simulink model "F16_openloop_linearization"  (R2018b)
settings: Solver=ode4  StartTime=0.0  StopTime=100.0  FixedStep=0.1  RelTol=1e-3  EnableMultiTasking=on
values from neighbouring files (symbols this model uses):
  fi_flag_Simulink = 0    [FindF16Dynamics.m]    (also in runF16model.m = 1)
libraries: simulink_extras x1
settings Model: Creator=Administrator  LastModifiedBy=LXS
settings DataIOCC: ExternalInput=[0 0.235629886402192 -0.0257557884830845 -0.00060101434994637 0.0105189516288919]  InitialState=[]  LimitDataPoints=on  LoadExternalInput=on  LoadInitialState=on  SaveFormat=Array  SignalLoggingSaveFormat=ModelDataLogs  SignalLoggingName=sigsOut
settings OptimizationCC: DefaultParameterBehavior=Inlined  BufferReuse=off  ExpressionDepthLimit=2147483647  InitFltsAndDblsToZero=on  LifeSpan=inf
settings DebuggingCC: SaveWithParameterizedLinksMsg=none  UnderspecifiedInitializationDetection=Classic  MergeDetectMultiDrivingBlocksExec=none  SignalResolutionControl=TryResolveAllWithWarning  MultiTaskDSMMsg=warning  MultiTaskCondExecSysMsg=none  FcnCallInpInsideContextMsg=warning  StateNameClashWarn=warning  InitInArrayFormatMsg=none  SFUnexpectedBacktrackingDiag=warning  SFNoUnconditionalDefaultTransitionDiag=warning  SFExecutionAtInitializationDiag=none
settings HardwareCC: ProdBitPerPointer=32  ProdBitPerSizeT=32  ProdBitPerPtrDiffT=32  ProdLargestAtomicFloat=None  ProdIntDivRoundTo=Undefined  ProdEndianess=Unspecified  ProdWordSize=32  ProdHWDeviceType=32-bit Generic  TargetUnknown=on
settings ModelReferenceCC: PropagateSignalLabelsOutOfModel=off
settings SFSimCC: SimUseLocalCustomCode=off
settings RTWCC: RTWUseLocalCustomCode=off
settings CodeAppCC: StateflowObjectComments=on
settings GRTTargetCC: TargetFcnLib=ansi_tfl_tmw.mat  TargetLangStandard=C89/C90 (ANSI)  GeneratePreprocessorConditionals=Disable all  CombineOutputUpdateFcns=off  GRTInterface=on
settings ConfigComp: CovMetricSettings=dw  CovHtmlReporting=on  CovSaveCumulativeToWorkspaceVar=on  CovSaveSingleToWorkspaceVar=on  CovExternalEMLEnable=off  CovSFcnEnable=off

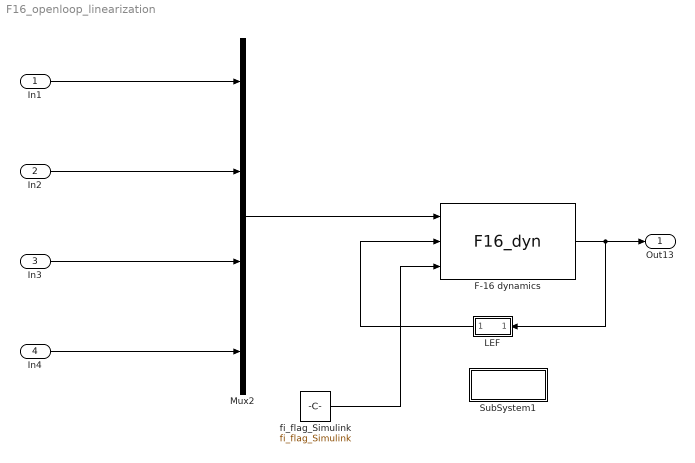
== system F16_openloop_linearization ==
  In1 : Inport
  In2 : Inport  Port=2
  In3 : Inport  Port=3
  In4 : Inport  Port=4
  F-16 dynamics : S-Function  FunctionName=F16_dyn  Parameters=init_x  SFunctionDeploymentMode=off  EnableBusSupport=off
      mask Display: image(imread('f16.jpg'))
  LEF : Subsystem
      mask Display: port_label('output', 1, 'dlef')
  Mux2 : Mux
  SubSystem1 : Subsystem
      settings: OpenFcn=edit(fullfile(cd,'F16_dyn.c'))
      mask Display: disp('F16_dyn.c');
  fi_flag_Simulink : Constant  Value=fi_flag_Simulink
  Out13 : Outport
  wires:
  F-16 dynamics/1 -> Out13/1, LEF/1(state)
  fi_flag_Simulink/1 -> F-16 dynamics/3
  LEF/1("delta_lef ") -> F-16 dynamics/2
  Mux2/1 -> F-16 dynamics/1
  In2/1 -> Mux2/2
  In3/1 -> Mux2/3
  In4/1 -> Mux2/4
  In1/1 -> Mux2/1

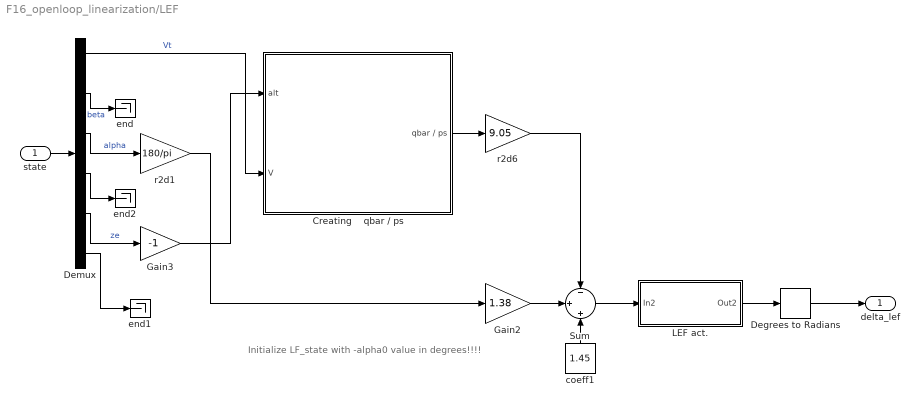
== system F16_openloop_linearization/LEF ==
  note: Initialize LF_state with -alpha0 value in degrees!!!!
  state : Inport
  Creating    qbar / ps : Subsystem
  Degrees to Radians : simulink_extras/Transformations/Degrees to Radians
  Demux : Demux  Outputs=[1 1 1 8 1 1]
  Gain2 : Gain  Gain=1.38  SaturateOnIntegerOverflow=on  OutDataTypeStr=Inherit: Same as input  ParamDataTypeStr=Inherit: Same as input
  Gain3 : Gain  Gain=-1  SaturateOnIntegerOverflow=on  OutDataTypeStr=Inherit: Same as input  ParamDataTypeStr=Inherit: Same as input
  LEF act. : Subsystem
  Sum : Sum  Inputs=-|+|+  SaturateOnIntegerOverflow=on  InputSameDT=on  OutDataTypeStr=Inherit: Same as first input
  coeff1 : Constant  Value=1.45
  end : Terminator
  end1 : Terminator
  end2 : Terminator
  r2d1 : Gain  Gain=180/pi  SaturateOnIntegerOverflow=on  OutDataTypeStr=Inherit: Same as input  ParamDataTypeStr=Inherit: Same as input
  r2d6 : Gain  Gain=9.05  SaturateOnIntegerOverflow=on  OutDataTypeStr=Inherit: Same as input  ParamDataTypeStr=Inherit: Same as input
  "delta_lef " : Outport
  wires:
  Degrees to Radians/1 -> "delta_lef "/1
  Gain3/1 -> Creating    qbar / ps/1(alt)
  Sum/1 -> LEF act./1(In2)
  state/1 -> Demux/1
  Gain2/1 -> Sum/2
  coeff1/1 -> Sum/3
  Creating    qbar / ps/1(qbar / ps) -> r2d6/1
  r2d6/1 -> Sum/1
  Demux/1 -> Creating    qbar / ps/2(V)  "Vt"
  Demux/2 -> end/1  "beta"
  Demux/3 -> r2d1/1  "alpha"
  Demux/4 -> end2/1
  Demux/5 -> Gain3/1  "ze"
  Demux/6 -> end1/1
  LEF act./1(Out2) -> Degrees to Radians/1
  r2d1/1 -> Gain2/1

== system F16_openloop_linearization/SubSystem1 ==

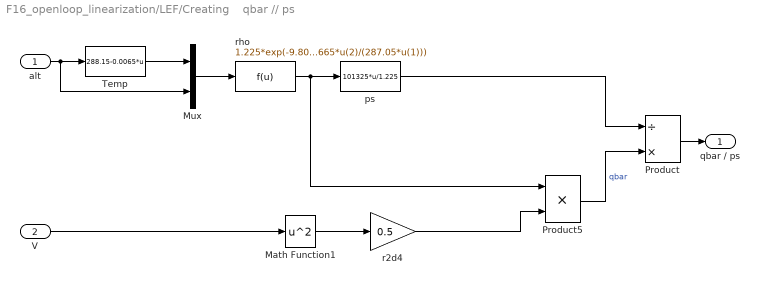
== system F16_openloop_linearization/LEF/Creating    qbar // ps ==
  alt : Inport
  V : Inport  Port=2
  Math Function1 : Math  Operator=square  SaturateOnIntegerOverflow=on
  Mux : Mux  Inputs=2
  Product : Product  Inputs=/*  SaturateOnIntegerOverflow=on  InputSameDT=on  OutDataTypeStr=Inherit: Same as first input
  Product5 : Product  Inputs=**  SaturateOnIntegerOverflow=on  InputSameDT=on  OutDataTypeStr=Inherit: Same as first input
  Temp : Fcn  Expr=288.15-0.0065*u
  ps : Fcn  Expr=101325*u/1.225
  r2d4 : Gain  Gain=0.5  SaturateOnIntegerOverflow=on  OutDataTypeStr=Inherit: Same as input  ParamDataTypeStr=Inherit: Same as input
  rho : Fcn  Expr=1.225*exp(-9.80665*u(2)/(287.05*u(1)))
  qbar / ps : Outport
  wires:
  ps/1 -> Product/1
  rho/1 -> Product5/1, ps/1
  Mux/1 -> rho/1
  Temp/1 -> Mux/1
  alt/1 -> Mux/2, Temp/1
  Math Function1/1 -> r2d4/1
  r2d4/1 -> Product5/2
  Product5/1 -> Product/2  "qbar"
  Product/1 -> qbar / ps/1
  V/1 -> Math Function1/1

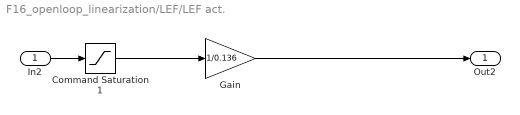
== system F16_openloop_linearization/LEF/LEF act. ==
  In2 : Inport
  Command Saturation1 : Saturate  UpperLimit=25  LowerLimit=0
  Gain : Gain  Gain=1/0.136  SaturateOnIntegerOverflow=on  OutDataTypeStr=Inherit: Same as input  ParamDataTypeStr=Inherit: Same as input
  Out2 : Outport
  wires:
  In2/1 -> Command Saturation1/1
  Command Saturation1/1 -> Gain/1
  Gain/1 -> Out2/1
